simulink model "sampleModel20"  (R2021a)
settings: Solver=VariableStepAuto  StartTime=0.0  StopTime=10.0  RelTol=1e-3
undefined symbols (not defined in the file): DiscIntNeverNeededParam, magnitude, Newton, Raphson
libraries: simulink x274, pid_lib x17
(part 15 of 16)

== system sampleModel20/cfblk94/cfblk8/cfblk9/cfblk5 ==
  cfblk1 : Inport
  cfblk6 : Inport  Port=2
  cfblk7 : Inport  Port=3
  cfblk8 : Inport  Port=4
  cfblk9 : Inport  Port=5
  cfblk10 : Inport  Port=6
  cfblk3 : Assignment  DiagnosticForDimensions=Warning  IndexOptions=Index vector (dialog)  Indices=1  OutputSizes=1
  cfblk4 : Sin  TimeSource=Use external signal  SampleTime=0
  cfblk5 : Sum  Inputs=+-
  cfblk2 : Outport
  cfblk11 : Outport  Port=2
  wires:
  cfblk10/1 -> cfblk4/1
  cfblk1/1 -> cfblk2/1
  cfblk8/1 -> cfblk11/1
  cfblk9/1 -> cfblk5/1
  cfblk4/1 -> cfblk3/1
  cfblk7/1 -> cfblk3/2
  cfblk3/1 -> cfblk5/2

== system sampleModel20/cfblk94/cfblk9/cfblk6/cfblk10 ==
  cfblk1 : Inport
  cfblk3 : Inport  Port=2
  cfblk4 : Inport  Port=3
  cfblk5 : Inport  Port=4
  cfblk6 : Inport  Port=5
  cfblk7 : Inport  Port=6
  cfblk8 : Inport  Port=7
  cfblk9 : Inport  Port=8
  cfblk10 : Inport  Port=9
  cfblk11 : Inport  Port=10
  cfblk2 : Outport
  cfblk12 : Outport  Port=2
  cfblk13 : Outport  Port=3
  cfblk14 : Outport  Port=4
  wires:
  cfblk10/1 -> cfblk2/1
  cfblk6/1 -> cfblk12/1
  cfblk11/1 -> cfblk14/1
  cfblk7/1 -> cfblk13/1

== system sampleModel20/cfblk94/cfblk9/cfblk6/cfblk8 ==
  cfblk1 : Inport
  cfblk9 : Inport  Port=2
  cfblk10 : Inport  Port=3
  cfblk11 : Inport  Port=4
  cfblk12 : Inport  Port=5
  cfblk14 : Delay  SampleTime=1
  cfblk3 : Sqrt  Operator=rSqrt  AlgorithmType=Newton-Raphson  SaturateOnIntegerOverflow=on
  cfblk4 : Product
  cfblk5 : Sum  Inputs=+-
  cfblk6 : Math  SaturateOnIntegerOverflow=on
  cfblk7 : Abs
  cfblk8 : Sum  Inputs=+-
  cfblk2 : Outport
  cfblk13 : Outport  Port=2
  wires:
  cfblk8/1 -> cfblk7/1
  cfblk6/1 -> cfblk5/2
  cfblk5/1 -> cfblk4/1
  cfblk1/1 -> cfblk6/1
  cfblk12/1 -> cfblk3/1
  cfblk10/1 -> cfblk4/2
  cfblk3/1 -> cfblk8/1
  cfblk11/1 -> cfblk8/2
  cfblk7/1 -> cfblk13/1
  cfblk9/1 -> cfblk2/1
  cfblk4/1 -> cfblk14/1
  cfblk14/1 -> cfblk5/1

== system sampleModel20/cfblk94/cfblk9/cfblk6/cfblk9 ==
  cfblk1 : Inport
  cfblk7 : Inport  Port=2
  cfblk8 : Inport  Port=3
  cfblk9 : Inport  Port=4
  cfblk12 : Delay  SampleTime=1
  cfblk3 : Assignment  DiagnosticForDimensions=Warning  IndexOptions=Index vector (dialog)  Indices=1  OutputSizes=1
  cfblk4 : DotProduct  InputSameDT=on  OutDataTypeStr=Inherit: Inherit via internal rule
  cfblk5 : Sum  Inputs=|++
  cfblk6 : Math  Operator=log  SaturateOnIntegerOverflow=on
  cfblk2 : Outport
  cfblk10 : Outport  Port=2
  cfblk11 : Outport  Port=3
  wires:
  cfblk9/1 -> cfblk6/1
  cfblk8/1 -> cfblk11/1
  cfblk5/1 -> cfblk10/1, cfblk4/2, cfblk3/2
  cfblk1/1 -> cfblk5/2
  cfblk6/1 -> cfblk4/1
  cfblk7/1 -> cfblk3/1
  cfblk4/1 -> cfblk2/1
  cfblk3/1 -> cfblk12/1
  cfblk12/1 -> cfblk5/1

== system sampleModel20/cfblk95/cfblk10/cfblk7/cfblk7 ==
  cfblk1 : Inport
  cfblk7 : Inport  Port=2
  cfblk3 : Sum  Inputs=+
  cfblk4 : MinMax
  cfblk5 : Sqrt  SaturateOnIntegerOverflow=on
  cfblk6 : Bias  Bias=[-377808434.956185]
  cfblk8 : Delay  SampleTime=1
  cfblk2 : Outport
  wires:
  cfblk6/1 -> cfblk4/1
  cfblk3/1 -> cfblk5/1
  cfblk1/1 -> cfblk2/1
  cfblk5/1 -> cfblk6/1
  cfblk4/1 -> cfblk8/1
  cfblk8/1 -> cfblk3/1

== system sampleModel20/cfblk95/cfblk10/cfblk7/cfblk8 ==
  cfblk1 : Inport
  cfblk6 : Inport  Port=2
  cfblk7 : Inport  Port=3
  cfblk8 : Inport  Port=4
  cfblk9 : Inport  Port=5
  cfblk10 : Delay  SampleTime=1
  cfblk3 : Gain  Gain=[-39886875.988626]
  cfblk4 : ComplexToMagnitudeAngle
  cfblk5 : Reshape
  cfblk2 : Outport
  wires:
  cfblk3/1 -> cfblk4/1
  cfblk4/2 -> cfblk5/1
  cfblk7/1 -> cfblk2/1
  cfblk4/1 -> cfblk10/1
  cfblk10/1 -> cfblk3/1

== system sampleModel20/cfblk95/cfblk10/cfblk7/cfblk9 ==
  cfblk1 : Inport
  cfblk8 : Inport  Port=2
  cfblk9 : Inport  Port=3
  cfblk10 : Inport  Port=4
  cfblk11 : Inport  Port=5
  cfblk13 : Delay  SampleTime=1
  cfblk3 : Product
  cfblk4 : Sin  TimeSource=Use external signal  SampleTime=0
  cfblk5 : simulink/Math Operations/Slider Gain  gain=1  low=0  high=2
  cfblk6 : simulink/Math Operations/Slider Gain  gain=1  low=0  high=2
  cfblk7 : Product
  cfblk2 : Outport
  cfblk12 : Outport  Port=2
  wires:
  cfblk10/1 -> cfblk3/1
  cfblk8/1 -> cfblk7/1
  cfblk3/1 -> cfblk2/1
  cfblk1/1 -> cfblk5/1
  cfblk4/1 -> cfblk7/2
  cfblk7/1 -> cfblk6/1
  cfblk11/1 -> cfblk3/2
  cfblk5/1 -> cfblk12/1
  cfblk6/1 -> cfblk13/1
  cfblk13/1 -> cfblk4/1

== system sampleModel20/cfblk95/cfblk11/cfblk5/cfblk7 ==
  cfblk1 : Inport
  cfblk7 : Inport  Port=2
  cfblk8 : Inport  Port=3
  cfblk9 : Inport  Port=4
  cfblk3 : ComplexToRealImag
  cfblk4 : Squeeze
  cfblk5 : UnaryMinus
  cfblk6 : Squeeze
  cfblk2 : Outport
  wires:
  cfblk1/1 -> cfblk2/1
  cfblk9/1 -> cfblk5/1
  cfblk8/1 -> cfblk6/1
  cfblk6/1 -> cfblk4/1
  cfblk5/1 -> cfblk3/1

== system sampleModel20/cfblk95/cfblk11/cfblk5/cfblk8 ==
  cfblk1 : Inport
  cfblk9 : Inport  Port=2
  cfblk10 : Inport  Port=3
  cfblk11 : Inport  Port=4
  cfblk12 : Inport  Port=5
  cfblk13 : Inport  Port=6
  cfblk16 : Delay  SampleTime=1
  cfblk3 : Product  Inputs=*
  cfblk4 : Assignment  DiagnosticForDimensions=Warning  IndexOptions=Index vector (dialog)  Indices=1  OutputSizes=1
  cfblk5 : UnaryMinus
  cfblk6 : MinMax  Inputs=3
  cfblk7 : Sqrt  SaturateOnIntegerOverflow=on
  cfblk8 : ComplexToRealImag
  cfblk2 : Outport
  cfblk14 : Outport  Port=2
  cfblk15 : Outport  Port=3
  wires:
  cfblk7/1 -> cfblk15/1
  cfblk11/1 -> cfblk14/1
  cfblk6/1 -> cfblk5/1
  cfblk8/1 -> cfblk4/1
  cfblk10/1 -> cfblk7/1
  cfblk8/2 -> cfblk6/1
  cfblk13/1 -> cfblk3/1
  cfblk1/1 -> cfblk4/2
  cfblk9/1 -> cfblk2/1
  cfblk3/1 -> cfblk8/1
  cfblk12/1 -> cfblk6/3
  cfblk5/1 -> cfblk16/1
  cfblk16/1 -> cfblk6/2

== system sampleModel20/cfblk95/cfblk11/cfblk5/cfblk9 ==
  cfblk1 : Inport
  cfblk8 : Inport  Port=2
  cfblk9 : Inport  Port=3
  cfblk10 : Inport  Port=4
  cfblk11 : Inport  Port=5
  cfblk3 : Sqrt  SaturateOnIntegerOverflow=on
  cfblk4 : Gain  Gain=[617379721.728358]
  cfblk5 : Reshape
  cfblk6 : simulink/Math Operations/MinMax Running Resettable  Function=min  vinit=0.0
  cfblk7 : Bias  Bias=[626466756.933337]
  cfblk2 : Outport
  cfblk12 : Outport  Port=2
  wires:
  cfblk4/1 -> cfblk5/1
  cfblk6/1 -> cfblk7/1
  cfblk11/1 -> cfblk2/1
  cfblk8/1 -> cfblk4/1
  cfblk5/1 -> cfblk3/1
  cfblk3/1 -> cfblk12/1
  cfblk9/1 -> cfblk6/1
  cfblk1/1 -> cfblk6/2

== system sampleModel20/cfblk95/cfblk11/cfblk6/cfblk3 ==
  cfblk1 : Inport
  cfblk9 : Inport  Port=2
  cfblk11 : Delay  SampleTime=1
  cfblk3 : Rounding
  cfblk4 : ComplexToRealImag
  cfblk5 : DotProduct  InputSameDT=on  OutDataTypeStr=Inherit: Inherit via internal rule
  cfblk6 : MinMax  Inputs=2
  cfblk7 : Sqrt  Operator=rSqrt  AlgorithmType=Newton-Raphson  SaturateOnIntegerOverflow=on
  cfblk8 : DotProduct  InputSameDT=on  OutDataTypeStr=Inherit: Inherit via internal rule
  cfblk2 : Outport
  cfblk10 : Outport  Port=2
  wires:
  cfblk9/1 -> cfblk4/1
  cfblk4/1 -> cfblk8/1
  cfblk8/1 -> cfblk6/2, cfblk11/1
  cfblk6/1 -> cfblk10/1
  cfblk5/1 -> cfblk8/2
  cfblk1/1 -> cfblk7/1
  cfblk7/1 -> cfblk3/1
  cfblk4/2 -> cfblk6/1, cfblk2/1
  cfblk3/1 -> cfblk5/2
  cfblk11/1 -> cfblk5/1

== system sampleModel20/cfblk95/cfblk11/cfblk6/cfblk4 ==
  cfblk1 : Inport
  cfblk7 : Inport  Port=2
  cfblk8 : Inport  Port=3
  cfblk9 : Inport  Port=4
  cfblk10 : Inport  Port=5
  cfblk14 : Delay  SampleTime=1
  cfblk3 : Product  Inputs=**
  cfblk4 : Math  Operator=hypot  SaturateOnIntegerOverflow=on
  cfblk5 : Squeeze
  cfblk6 : Sum  Inputs=+-
  cfblk2 : Outport
  cfblk11 : Outport  Port=2
  cfblk12 : Outport  Port=3
  cfblk13 : Outport  Port=4
  wires:
  cfblk4/1 -> cfblk5/1
  cfblk6/1 -> cfblk12/1
  cfblk10/1 -> cfblk3/1, cfblk4/1
  cfblk5/1 -> cfblk13/1, cfblk14/1
  cfblk1/1 -> cfblk2/1
  cfblk8/1 -> cfblk11/1
  cfblk7/1 -> cfblk3/2
  cfblk9/1 -> cfblk6/1
  cfblk3/1 -> cfblk6/2
  cfblk14/1 -> cfblk4/2

== system sampleModel20/cfblk95/cfblk6/cfblk5/cfblk10 ==
  cfblk1 : Inport
  cfblk8 : Inport  Port=2
  cfblk9 : Inport  Port=3
  cfblk3 : Sum  Inputs=+
  cfblk4 : Sqrt  SaturateOnIntegerOverflow=on
  cfblk5 : Trigonometry
  cfblk6 : Product  Inputs=*
  cfblk7 : Constant  Value=[-128317265.699425]  SampleTime=1
  cfblk2 : Outport
  cfblk10 : Outport  Port=2
  cfblk11 : Outport  Port=3
  cfblk12 : Outport  Port=4
  cfblk13 : Outport  Port=5
  cfblk14 : Outport  Port=6
  wires:
  cfblk7/1 -> cfblk12/1
  cfblk1/1 -> cfblk10/1, cfblk11/1
  cfblk9/1 -> cfblk13/1
  cfblk8/1 -> cfblk4/1
  cfblk6/1 -> cfblk14/1
  cfblk4/1 -> cfblk3/1
  cfblk5/1 -> cfblk2/1, cfblk6/1
  cfblk3/1 -> cfblk5/1

== system sampleModel20/cfblk95/cfblk6/cfblk5/cfblk8 ==
  cfblk1 : Inport
  cfblk10 : Inport  Port=2
  cfblk11 : Inport  Port=3
  cfblk12 : Inport  Port=4
  cfblk13 : Inport  Port=5
  cfblk14 : Inport  Port=6
  cfblk15 : Inport  Port=7
  cfblk16 : Inport  Port=8
  cfblk3 : Math  Operator=conj  SaturateOnIntegerOverflow=on
  cfblk4 : Sin  TimeSource=Use external signal  SampleTime=0
  cfblk5 : simulink/Math Operations/Slider Gain  gain=1  low=0  high=2
  cfblk6 : ComplexToRealImag
  cfblk7 : Sum  Inputs=+-
  cfblk8 : Sqrt  SaturateOnIntegerOverflow=on
  cfblk9 : Squeeze
  cfblk2 : Outport
  cfblk17 : Outport  Port=2
  wires:
  cfblk1/1 -> cfblk3/1
  cfblk12/1 -> cfblk8/1
  cfblk16/1 -> cfblk4/1
  cfblk15/1 -> cfblk5/1
  cfblk4/1 -> cfblk9/1
  cfblk10/1 -> cfblk6/1
  cfblk11/1 -> cfblk2/1
  cfblk7/1 -> cfblk17/1
  cfblk9/1 -> cfblk7/1
  cfblk8/1 -> cfblk7/2

== system sampleModel20/cfblk95/cfblk6/cfblk5/cfblk9 ==
  cfblk1 : Inport
  cfblk10 : Inport  Port=2
  cfblk11 : Inport  Port=3
  cfblk12 : Inport  Port=4
  cfblk13 : Inport  Port=5
  cfblk14 : Inport  Port=6
  cfblk15 : Inport  Port=7
  cfblk3 : Reshape
  cfblk4 : simulink/Math Operations/Slider Gain  gain=1  low=0  high=2
  cfblk5 : Reshape
  cfblk6 : UnaryMinus
  cfblk7 : Sum  Inputs=|++
  cfblk8 : Abs
  cfblk9 : simulink/Math Operations/MinMax Running Resettable  Function=min  vinit=0.0
  cfblk2 : Outport
  cfblk16 : Outport  Port=2
  cfblk17 : Outport  Port=3
  wires:
  cfblk11/1 -> cfblk9/1
  cfblk8/1 -> cfblk6/1
  cfblk3/1 -> cfblk8/1
  cfblk4/1 -> cfblk5/1
  cfblk7/1 -> cfblk4/1
  cfblk1/1 -> cfblk7/1
  cfblk15/1 -> cfblk9/2
  cfblk10/1 -> cfblk17/1
  cfblk14/1 -> cfblk7/2
  cfblk13/1 -> cfblk16/1
  cfblk6/1 -> cfblk2/1
  cfblk9/1 -> cfblk3/1

== system sampleModel20/cfblk95/cfblk6/cfblk6/cfblk10 ==
  cfblk1 : Inport
  cfblk6 : Inport  Port=2
  cfblk7 : Inport  Port=3
  cfblk8 : Inport  Port=4
  cfblk9 : Inport  Port=5
  cfblk10 : Inport  Port=6
  cfblk3 : DiscreteFir  SampleTime=1
  cfblk4 : UnaryMinus
  cfblk5 : Sum  Inputs=|++
  cfblk2 : Outport
  cfblk11 : Outport  Port=2
  wires:
  cfblk7/1 -> cfblk5/1
  cfblk9/1 -> cfblk2/1
  cfblk3/1 -> cfblk4/1
  cfblk6/1 -> cfblk5/2
  cfblk1/1 -> cfblk3/1
  cfblk5/1 -> cfblk11/1

== system sampleModel20/cfblk95/cfblk6/cfblk6/cfblk8 ==
  cfblk1 : Inport
  cfblk7 : Inport  Port=2
  cfblk8 : Inport  Port=3
  cfblk9 : Inport  Port=4
  cfblk10 : Delay  SampleTime=1
  cfblk3 : DiscreteTransferFcn  SampleTime=1
  cfblk4 : Sum  Inputs=+-
  cfblk5 : Gain  Gain=[-981035037.304290]
  cfblk6 : Product  Inputs=**
  cfblk2 : Outport
  wires:
  cfblk9/1 -> cfblk2/1
  cfblk6/1 -> cfblk5/1
  cfblk8/1 -> cfblk4/1
  cfblk3/1 -> cfblk6/1
  cfblk7/1 -> cfblk6/2
  cfblk1/1 -> cfblk4/2
  cfblk5/1 -> cfblk10/1
  cfblk10/1 -> cfblk3/1

== system sampleModel20/cfblk95/cfblk6/cfblk6/cfblk9 ==
  cfblk1 : Inport
  cfblk9 : Inport  Port=2
  cfblk10 : Inport  Port=3
  cfblk11 : Inport  Port=4
  cfblk12 : Inport  Port=5
  cfblk3 : Gain  Gain=[466248434.807061]
  cfblk4 : Trigonometry
  cfblk5 : Signum
  cfblk6 : Rounding
  cfblk7 : Squeeze
  cfblk8 : Sum  Inputs=+
  cfblk2 : Outport
  cfblk13 : Outport  Port=2
  wires:
  cfblk4/1 -> cfblk2/1
  cfblk9/1 -> cfblk6/1
  cfblk6/1 -> cfblk3/1
  cfblk10/1 -> cfblk4/1
  cfblk3/1 -> cfblk5/1
  cfblk1/1 -> cfblk7/1
  cfblk11/1 -> cfblk8/1
  cfblk12/1 -> cfblk13/1

== system sampleModel20/cfblk95/cfblk6/cfblk7/cfblk10 ==
  cfblk1 : Inport
  cfblk10 : Inport  Port=2
  cfblk11 : Inport  Port=3
  cfblk12 : Inport  Port=4
  cfblk13 : Inport  Port=5
  cfblk14 : Inport  Port=6
  cfblk15 : Inport  Port=7
  cfblk3 : Sqrt  Operator=rSqrt  AlgorithmType=Newton-Raphson  SaturateOnIntegerOverflow=on
  cfblk4 : Sum  Inputs=|++
  cfblk5 : Sum  Inputs=+
  cfblk6 : Signum
  cfblk7 : Gain  Gain=[306381383.293129]
  cfblk8 : Gain  Gain=[360787221.537150]
  cfblk9 : Polyval  Coefs=[ +2.081618890e-019, -1.441693666e-014, +4.719686976e-010, -8.536869453e-006, +1.621573104e-001, -8.087801117e+001 ]
  cfblk2 : Outport
  cfblk16 : Outport  Port=2
  wires:
  cfblk11/1 -> cfblk7/1
  cfblk15/1 -> cfblk3/1
  cfblk7/1 -> cfblk5/1
  cfblk14/1 -> cfblk8/1
  cfblk9/1 -> cfblk4/1
  cfblk1/1 -> cfblk9/1
  cfblk3/1 -> cfblk16/1
  cfblk13/1 -> cfblk6/1
  cfblk6/1 -> cfblk4/2
  cfblk4/1 -> cfblk2/1

== system sampleModel20/cfblk95/cfblk6/cfblk7/cfblk11 ==
  cfblk1 : Inport
  cfblk5 : Inport  Port=2
  cfblk6 : Inport  Port=3
  cfblk7 : Inport  Port=4
  cfblk8 : Inport  Port=5
  cfblk9 : Inport  Port=6
  cfblk3 : DiscreteFir  SampleTime=1
  cfblk4 : Sum  Inputs=-+
  cfblk2 : Outport
  cfblk10 : Outport  Port=2
  wires:
  cfblk8/1 -> cfblk10/1
  cfblk6/1 -> cfblk2/1
  cfblk5/1 -> cfblk3/1
  cfblk1/1 -> cfblk4/1
  cfblk7/1 -> cfblk4/2

== system sampleModel20/cfblk95/cfblk6/cfblk7/cfblk9 ==
  cfblk1 : Inport
  cfblk5 : Inport  Port=2
  cfblk6 : Inport  Port=3
  cfblk7 : Inport  Port=4
  cfblk3 : Sqrt  Operator=rSqrt  AlgorithmType=Newton-Raphson  SaturateOnIntegerOverflow=on
  cfblk4 : Squeeze
  cfblk2 : Outport
  wires:
  cfblk3/1 -> cfblk4/1
  cfblk1/1 -> cfblk3/1
  cfblk6/1 -> cfblk2/1

== system sampleModel20/cfblk95/cfblk7/cfblk4/cfblk10 ==
  cfblk1 : Inport
  cfblk8 : Inport  Port=2
  cfblk9 : Inport  Port=3
  cfblk10 : Inport  Port=4
  cfblk11 : Inport  Port=5
  cfblk12 : Inport  Port=6
  cfblk13 : Inport  Port=7
  cfblk3 : DiscreteZeroPole  Poles=[0 0.5]  Gain=1
  cfblk4 : Signum
  cfblk5 : Signum
  cfblk6 : simulink/Math Operations/Slider Gain  gain=1  low=0  high=2
  cfblk7 : Assignment  DiagnosticForDimensions=Warning  IndexOptions=Index vector (dialog)  Indices=1  OutputSizes=1
  cfblk2 : Outport
  cfblk14 : Outport  Port=2
  cfblk15 : Outport  Port=3
  cfblk16 : Outport  Port=4
  cfblk17 : Outport  Port=5
  wires:
  cfblk1/1 -> cfblk3/1
  cfblk7/1 -> cfblk16/1
  cfblk12/1 -> cfblk4/1
  cfblk3/1 -> cfblk5/1
  cfblk6/1 -> cfblk14/1
  cfblk11/1 -> cfblk15/1
  cfblk13/1 -> cfblk6/1
  cfblk8/1 -> cfblk2/1
  cfblk10/1 -> cfblk7/1
  cfblk5/1 -> cfblk17/1
  cfblk9/1 -> cfblk7/2

== system sampleModel20/cfblk95/cfblk7/cfblk4/cfblk7 ==
  cfblk1 : Inport
  cfblk7 : Inport  Port=2
  cfblk8 : Inport  Port=3
  cfblk9 : Inport  Port=4
  cfblk10 : Inport  Port=5
  cfblk11 : Inport  Port=6
  cfblk3 : DotProduct  InputSameDT=on  OutDataTypeStr=Inherit: Inherit via internal rule
  cfblk4 : ComplexToMagnitudeAngle
  cfblk5 : Sqrt  SaturateOnIntegerOverflow=on
  cfblk6 : Bias  Bias=[-832558987.435364]
  cfblk2 : Outport
  wires:
  cfblk11/1 -> cfblk6/1
  cfblk9/1 -> cfblk5/1
  cfblk5/1 -> cfblk3/1
  cfblk6/1 -> cfblk4/1
  cfblk7/1 -> cfblk2/1
  cfblk1/1 -> cfblk3/2

== system sampleModel20/cfblk95/cfblk7/cfblk4/cfblk8 ==
  cfblk1 : Inport
  cfblk8 : Inport  Port=2
  cfblk9 : Inport  Port=3
  cfblk10 : Inport  Port=4
  cfblk12 : Delay  SampleTime=1
  cfblk3 : Product  Inputs=**
  cfblk4 : Product  Inputs=*
  cfblk5 : Assignment  DiagnosticForDimensions=Warning  IndexOptions=Index vector (dialog)  Indices=1  OutputSizes=1
  cfblk6 : Signum
  cfblk7 : ComplexToRealImag
  cfblk2 : Outport
  cfblk11 : Outport  Port=2
  wires:
  cfblk3/1 -> cfblk5/1
  cfblk7/1 -> cfblk2/1
  cfblk8/1 -> cfblk7/1
  cfblk4/1 -> cfblk6/1
  cfblk10/1 -> cfblk5/2
  cfblk6/1 -> cfblk3/1
  cfblk7/2 -> cfblk11/1
  cfblk9/1 -> cfblk4/1
  cfblk5/1 -> cfblk12/1
  cfblk12/1 -> cfblk3/2

== system sampleModel20/cfblk95/cfblk7/cfblk4/cfblk9 ==
  cfblk1 : Inport
  cfblk8 : Inport  Port=2
  cfblk9 : Inport  Port=3
  cfblk10 : Inport  Port=4
  cfblk11 : Inport  Port=5
  cfblk12 : Inport  Port=6
  cfblk13 : Inport  Port=7
  cfblk14 : Inport  Port=8
  cfblk15 : Inport  Port=9
  cfblk3 : Product
  cfblk4 : Squeeze
  cfblk5 : Gain  Gain=[-607601415.190912]
  cfblk6 : Sqrt  Operator=rSqrt  AlgorithmType=Newton-Raphson  SaturateOnIntegerOverflow=on
  cfblk7 : Sum  Inputs=|++
  cfblk2 : Outport
  cfblk16 : Outport  Port=2
  cfblk17 : Outport  Port=3
  wires:
  cfblk13/1 -> cfblk3/1
  cfblk1/1 -> cfblk2/1
  cfblk5/1 -> cfblk4/1
  cfblk8/1 -> cfblk3/2
  cfblk3/1 -> cfblk16/1
  cfblk12/1 -> cfblk7/1
  cfblk11/1 -> cfblk6/1
  cfblk10/1 -> cfblk5/1
  cfblk15/1 -> cfblk7/2
  cfblk6/1 -> cfblk17/1

== system sampleModel20/cfblk95/cfblk7/cfblk5/cfblk5 ==
  cfblk1 : Inport
  cfblk8 : Inport  Port=2
  cfblk9 : Inport  Port=3
  cfblk10 : Inport  Port=4
  cfblk11 : Inport  Port=5
  cfblk12 : Inport  Port=6
  cfblk13 : Inport  Port=7
  cfblk3 : Trigonometry
  cfblk4 : Rounding
  cfblk5 : Product  Inputs=*
  cfblk6 : Sum  Inputs=+
  cfblk7 : Bias  Bias=[7544371.350967]
  cfblk2 : Outport
  cfblk14 : Outport  Port=2
  cfblk15 : Outport  Port=3
  wires:
  cfblk1/1 -> cfblk5/1
  cfblk10/1 -> cfblk2/1
  cfblk3/1 -> cfblk7/1
  cfblk9/1 -> cfblk6/1
  cfblk8/1 -> cfblk14/1
  cfblk11/1 -> cfblk3/1
  cfblk13/1 -> cfblk4/1
  cfblk4/1 -> cfblk15/1

== system sampleModel20/cfblk95/cfblk7/cfblk5/cfblk6 ==
  cfblk1 : Inport
  cfblk5 : Inport  Port=2
  cfblk6 : Inport  Port=3
  cfblk7 : Inport  Port=4
  cfblk3 : Product  Inputs=**
  cfblk4 : UnaryMinus
  cfblk2 : Outport
  cfblk8 : Outport  Port=2
  wires:
  cfblk5/1 -> cfblk4/1
  cfblk3/1 -> cfblk8/1
  cfblk1/1 -> cfblk2/1
  cfblk7/1 -> cfblk3/1
  cfblk6/1 -> cfblk3/2

== system sampleModel20/cfblk95/cfblk8/cfblk5/cfblk6 ==
  cfblk1 : Inport
  cfblk6 : Inport  Port=2
  cfblk7 : Inport  Port=3
  cfblk8 : Inport  Port=4
  cfblk3 : Sum  Inputs=|++
  cfblk4 : Gain  Gain=[-834854673.275591]
  cfblk5 : Sum  Inputs=+-
  cfblk2 : Outport
  cfblk9 : Outport  Port=2
  cfblk10 : Outport  Port=3
  wires:
  cfblk7/1 -> cfblk3/1
  cfblk3/1 -> cfblk10/1
  cfblk5/1 -> cfblk3/2
  cfblk8/1 -> cfblk9/1
  cfblk1/1 -> cfblk2/1
  cfblk6/1 -> cfblk4/1, cfblk5/2
  cfblk4/1 -> cfblk5/1

== system sampleModel20/cfblk95/cfblk8/cfblk6/cfblk10 ==
  cfblk1 : Inport
  cfblk5 : Inport  Port=2
  cfblk6 : Inport  Port=3
  cfblk7 : Inport  Port=4
  cfblk8 : Inport  Port=5
  cfblk3 : Sqrt  Operator=rSqrt  AlgorithmType=Newton-Raphson  SaturateOnIntegerOverflow=on
  cfblk4 : Sum  Inputs=+-
  cfblk2 : Outport
  wires:
  cfblk6/1 -> cfblk3/1
  cfblk7/1 -> cfblk2/1
  cfblk1/1 -> cfblk4/1
  cfblk8/1 -> cfblk4/2

== system sampleModel20/cfblk95/cfblk8/cfblk6/cfblk11 ==
  cfblk1 : Inport
  cfblk4 : Inport  Port=2
  cfblk5 : Inport  Port=3
  cfblk6 : Inport  Port=4
  cfblk3 : Sqrt  SaturateOnIntegerOverflow=on
  cfblk2 : Outport
  cfblk7 : Outport  Port=2
  wires:
  cfblk1/1 -> cfblk3/1
  cfblk4/1 -> cfblk7/1
  cfblk5/1 -> cfblk2/1

== system sampleModel20/cfblk95/cfblk8/cfblk6/cfblk12 ==
  cfblk1 : Inport
  cfblk9 : Inport  Port=2
  cfblk10 : Inport  Port=3
  cfblk11 : Inport  Port=4
  cfblk12 : Inport  Port=5
  cfblk13 : Inport  Port=6
  cfblk14 : Delay  SampleTime=1
  cfblk3 : MinMax  Function=max
  cfblk4 : PermuteDimensions
  cfblk5 : Sin  TimeSource=Use external signal  SampleTime=0
  cfblk6 : PermuteDimensions
  cfblk7 : Product
  cfblk8 : DotProduct  InputSameDT=on  OutDataTypeStr=Inherit: Inherit via internal rule
  cfblk2 : Outport
  wires:
  cfblk8/1 -> cfblk4/1
  cfblk11/1 -> cfblk2/1
  cfblk13/1 -> cfblk7/1
  cfblk5/1 -> cfblk6/1
  cfblk1/1 -> cfblk8/1
  cfblk12/1 -> cfblk7/2
  cfblk10/1 -> cfblk8/2
  cfblk7/1 -> cfblk3/1
  cfblk6/1 -> cfblk14/1
  cfblk14/1 -> cfblk5/1

== system sampleModel20/cfblk95/cfblk8/cfblk6/cfblk7 ==
  cfblk1 : Inport
  cfblk5 : Inport  Port=2
  cfblk6 : Inport  Port=3
  cfblk7 : Inport  Port=4
  cfblk3 : pid_lib/PID Controller (2DOF)  Controller=PID  Form=Parallel  TimeDomain=Discrete-time  UseExternalTs=off  SampleTime=1  IntegratorMethod=Forward Euler  FilterMethod=Forward Euler  ControllerParametersSource=internal  P=1  I=1  D=0  UseFilter=on  N=100  b=1  c=1  TunerSelectOption=Transfer Function Based (PID Tuner App)  InitialConditionSource=internal  InitialConditionForIntegrator=0  InitialConditionForFilter=0  DifferentiatorICPrevScaledInput=0  ExternalReset=none  TrackingMode=off  Kt=1  LimitOutput=off  SatLimitsSource=internal  UpperSaturationLimit=inf  LowerSaturationLimit=-inf  LinearizeAsGain=off  AntiWindupMode=none  Kb=1  POutMin=[]  POutMax=[]  IOutMin=[]  IOutMax=[]  DOutMin=[]  DOutMax=[]  NOutMin=[]  NOutMax=[]  bOutMin=[]  bOutMax=[]  cOutMin=[]  cOutMax=[]  SumOutMin=[]  SumOutMax=[]  SaturationOutMin=[]  SaturationOutMax=[]  PParamMin=[]  PParamMax=[]  IParamMin=[]  IParamMax=[]  DParamMin=[]  DParamMax=[]  NParamMin=[]  NParamMax=[]  bParamMin=[]  bParamMax=[]  cParamMin=[]  cParamMax=[]  KbParamMin=[]  KbParamMax=[]  KtParamMin=[]  KtParamMax=[]  KbOutMin=[]  KbOutMax=[]  KtOutMin=[]  KtOutMax=[]  IntegratorOutMin=[]  IntegratorOutMax=[]  FilterOutMin=[]  FilterOutMax=[]  SumI1OutMin=[]  SumI1OutMax=[]  SumI2OutMin=[]  SumI2OutMax=[]  SumI3OutMin=[]  SumI3OutMax=[]  SumI4OutMin=[]  SumI4OutMax=[]  SumDOutMin=[]  SumDOutMax=[]  Sum1OutMin=[]  Sum1OutMax=[]  Sum2OutMin=[]  Sum2OutMax=[]  Sum3OutMin=[]  Sum3OutMax=[]  DifferentiatorOutMin=[]  DifferentiatorOutMax=[]  FilterDiffOutCoefMin=[]  FilterDiffOutCoefMax=[]  ReciprocalOutMin=[]  ReciprocalOutMax=[]  SumDenOutMin=[]  SumDenOutMax=[]  SumNumOutMin=[]  SumNumOutMax=[]  DivideOutMin=[]  DivideOutMax=[]  UdiffTsProdOutMin=[]  UdiffTsProdOutMax=[]  NTsProdOutMin=[]  NTsProdOutMax=[]  UintegralTsProdOutMin=[]  UintegralTsProdOutMax=[]  UngainTsProdOutMin=[]  UngainTsProdOutMax=[]  IntegratorContinuousStateAttributes=''  IntegratorStateMustResolveToSignalObject=off  IntegratorRTWStateStorageClass=Auto  FilterContinuousStateAttributes=''  FilterStateMustResolveToSignalObject=off  FilterRTWStateStorageClass=Auto  ParallelPVariant=InternalParameters  IdealPVariant=Disabled  IVariant=InternalParameters  DVariant=InternalParameters  bVariant=InternalParameters  cVariant=InternalParameters  IntegratorVariant=Discrete  SatVariant=Disabled  AWVariant=Passthrough  PCopyVariant=Disabled  TRVariant=Disabled  FdbkBlocksVariant=Forward  IdealPFdbkVariant=Disabled  SatFdbkVariant=Disabled  DerivativeFilterVariant=ForwardEulerFilter  NVariant=InternalParameters  NCopyVariant=Disabled  FilterICVariant=InternalICsFilter  IntegratorICVariant=InternalICs  ExternalResetVariant=Disabled  TRSumVariant=Passthrough  SumFdbkVariant=Disabled  SumVariant=Sum_PID  TsampFilterVariant=InternalTs  TsampNgainVariant=Passthrough  TsampIntegralVariant=Passthrough  ExternalSaturationOutDataTypeStr=Inherit: Same as second input
      settings: SourceProductBaseCode=SL
  cfblk4 : Sqrt  Operator=rSqrt  AlgorithmType=Newton-Raphson  SaturateOnIntegerOverflow=on
  cfblk2 : Outport
  cfblk8 : Outport  Port=2
  cfblk9 : Outport  Port=3
  wires:
  cfblk6/1 -> cfblk4/1
  cfblk7/1 -> cfblk9/1
  cfblk4/1 -> cfblk2/1
  cfblk1/1 -> cfblk3/1
  cfblk3/1 -> cfblk8/1
  cfblk5/1 -> cfblk3/2

== system sampleModel20/cfblk95/cfblk8/cfblk6/cfblk8 ==
  cfblk1 : Inport
  cfblk10 : Inport  Port=2
  cfblk11 : Inport  Port=3
  cfblk12 : Inport  Port=4
  cfblk13 : Inport  Port=5
  cfblk14 : Inport  Port=6
  cfblk15 : Inport  Port=7
  cfblk3 : simulink/Discrete/Difference  ICPrevInput=0.0  OutMin=[]  OutMax=[]  OutDataTypeStr=Inherit: Inherit via back propagation  OutDataType=fixdt(1, 16)  OutScaling=2^-10  DoSatur=off
  cfblk4 : DotProduct  InputSameDT=on  OutDataTypeStr=Inherit: Inherit via internal rule
  cfblk5 : Reshape
  cfblk6 : simulink/Math Operations/Slider Gain  gain=1  low=0  high=2
  cfblk7 : Sin  TimeSource=Use external signal  SampleTime=0
  cfblk8 : UnaryMinus
  cfblk9 : Abs
  cfblk2 : Outport
  wires:
  cfblk3/1 -> cfblk6/1
  cfblk13/1 -> cfblk2/1
  cfblk7/1 -> cfblk9/1
  cfblk1/1 -> cfblk5/1
  cfblk9/1 -> cfblk8/1
  cfblk6/1 -> cfblk7/1
  cfblk11/1 -> cfblk3/1
  cfblk14/1 -> cfblk4/1
  cfblk15/1 -> cfblk4/2

== system sampleModel20/cfblk95/cfblk8/cfblk6/cfblk9 ==
  cfblk1 : Inport
  cfblk8 : Inport  Port=2
  cfblk9 : Inport  Port=3
  cfblk12 : Delay  SampleTime=1
  cfblk13 : Delay  SampleTime=1
  cfblk3 : DiscreteStateSpace
  cfblk4 : simulink/Math Operations/MinMax Running Resettable  Function=min  vinit=0.0
  cfblk5 : Product  Inputs=**
  cfblk6 : Gain  Gain=[-761792145.113436]
  cfblk7 : Sum  Inputs=+
  cfblk2 : Outport
  cfblk10 : Outport  Port=2
  cfblk11 : Outport  Port=3
  wires:
  cfblk4/1 -> cfblk10/1, cfblk5/2
  cfblk5/1 -> cfblk6/1, cfblk13/1
  cfblk8/1 -> cfblk11/1
  cfblk9/1 -> cfblk3/1
  cfblk6/1 -> cfblk7/1
  cfblk3/1 -> cfblk2/1
  cfblk1/1 -> cfblk4/1
  cfblk7/1 -> cfblk12/1
  cfblk12/1 -> cfblk5/1
  cfblk13/1 -> cfblk4/2

== system sampleModel20/cfblk95/cfblk8/cfblk7/cfblk5 ==
  cfblk1 : Inport
  cfblk6 : Inport  Port=2
  cfblk7 : Inport  Port=3
  cfblk8 : Inport  Port=4
  cfblk9 : Inport  Port=5
  cfblk10 : Inport  Port=6
  cfblk3 : Sum  Inputs=+-
  cfblk4 : Sum  Inputs=|++
  cfblk5 : Product
  cfblk2 : Outport
  wires:
  cfblk10/1 -> cfblk4/1
  cfblk9/1 -> cfblk3/1
  cfblk5/1 -> cfblk2/1
  cfblk1/1 -> cfblk3/2
  cfblk8/1 -> cfblk5/1
  cfblk3/1 -> cfblk4/2
  cfblk6/1 -> cfblk5/2

== system sampleModel20/cfblk95/cfblk8/cfblk7/cfblk6 ==
  cfblk1 : Inport
  cfblk12 : Inport  Port=2
  cfblk13 : Inport  Port=3
  cfblk14 : Inport  Port=4
  cfblk10 : Product  Inputs=*
  cfblk11 : Sin  TimeSource=Use external signal  SampleTime=0
  cfblk17 : Delay  SampleTime=1
  cfblk3 : Signum
  cfblk4 : Sum  Inputs=|++
  cfblk5 : Sum  Inputs=+
  cfblk6 : Sqrt  SaturateOnIntegerOverflow=on
  cfblk7 : Abs
  cfblk8 : Math  Operator=mod  SaturateOnIntegerOverflow=on
  cfblk9 : Trigonometry
  cfblk2 : Outport
  cfblk15 : Outport  Port=2
  cfblk16 : Outport  Port=3
  wires:
  cfblk10/1 -> cfblk8/1, cfblk2/1
  cfblk1/1 -> cfblk6/1
  cfblk8/1 -> cfblk4/1
  cfblk9/1 -> cfblk4/2
  cfblk14/1 -> cfblk10/1
  cfblk13/1 -> cfblk16/1
  cfblk12/1 -> cfblk3/1
  cfblk4/1 -> cfblk15/1
  cfblk7/1 -> cfblk9/1
  cfblk6/1 -> cfblk8/2
  cfblk5/1 -> cfblk11/1
  cfblk3/1 -> cfblk7/1
  cfblk11/1 -> cfblk17/1
  cfblk17/1 -> cfblk5/1

== system sampleModel20/cfblk95/cfblk8/cfblk7/cfblk7 ==
  cfblk1 : Inport
  cfblk9 : Inport  Port=2
  cfblk10 : Inport  Port=3
  cfblk11 : Inport  Port=4
  cfblk12 : Inport  Port=5
  cfblk13 : Inport  Port=6
  cfblk17 : Delay  SampleTime=1
  cfblk3 : pid_lib/PID Controller (2DOF)  Controller=PID  Form=Parallel  TimeDomain=Discrete-time  UseExternalTs=off  SampleTime=1  IntegratorMethod=Forward Euler  FilterMethod=Forward Euler  ControllerParametersSource=internal  P=1  I=1  D=0  UseFilter=on  N=100  b=1  c=1  TunerSelectOption=Transfer Function Based (PID Tuner App)  InitialConditionSource=internal  InitialConditionForIntegrator=0  InitialConditionForFilter=0  DifferentiatorICPrevScaledInput=0  ExternalReset=none  TrackingMode=off  Kt=1  LimitOutput=off  SatLimitsSource=internal  UpperSaturationLimit=inf  LowerSaturationLimit=-inf  LinearizeAsGain=off  AntiWindupMode=none  Kb=1  POutMin=[]  POutMax=[]  IOutMin=[]  IOutMax=[]  DOutMin=[]  DOutMax=[]  NOutMin=[]  NOutMax=[]  bOutMin=[]  bOutMax=[]  cOutMin=[]  cOutMax=[]  SumOutMin=[]  SumOutMax=[]  SaturationOutMin=[]  SaturationOutMax=[]  PParamMin=[]  PParamMax=[]  IParamMin=[]  IParamMax=[]  DParamMin=[]  DParamMax=[]  NParamMin=[]  NParamMax=[]  bParamMin=[]  bParamMax=[]  cParamMin=[]  cParamMax=[]  KbParamMin=[]  KbParamMax=[]  KtParamMin=[]  KtParamMax=[]  KbOutMin=[]  KbOutMax=[]  KtOutMin=[]  KtOutMax=[]  IntegratorOutMin=[]  IntegratorOutMax=[]  FilterOutMin=[]  FilterOutMax=[]  SumI1OutMin=[]  SumI1OutMax=[]  SumI2OutMin=[]  SumI2OutMax=[]  SumI3OutMin=[]  SumI3OutMax=[]  SumI4OutMin=[]  SumI4OutMax=[]  SumDOutMin=[]  SumDOutMax=[]  Sum1OutMin=[]  Sum1OutMax=[]  Sum2OutMin=[]  Sum2OutMax=[]  Sum3OutMin=[]  Sum3OutMax=[]  DifferentiatorOutMin=[]  DifferentiatorOutMax=[]  FilterDiffOutCoefMin=[]  FilterDiffOutCoefMax=[]  ReciprocalOutMin=[]  ReciprocalOutMax=[]  SumDenOutMin=[]  SumDenOutMax=[]  SumNumOutMin=[]  SumNumOutMax=[]  DivideOutMin=[]  DivideOutMax=[]  UdiffTsProdOutMin=[]  UdiffTsProdOutMax=[]  NTsProdOutMin=[]  NTsProdOutMax=[]  UintegralTsProdOutMin=[]  UintegralTsProdOutMax=[]  UngainTsProdOutMin=[]  UngainTsProdOutMax=[]  IntegratorContinuousStateAttributes=''  IntegratorStateMustResolveToSignalObject=off  IntegratorRTWStateStorageClass=Auto  FilterContinuousStateAttributes=''  FilterStateMustResolveToSignalObject=off  FilterRTWStateStorageClass=Auto  ParallelPVariant=InternalParameters  IdealPVariant=Disabled  IVariant=InternalParameters  DVariant=InternalParameters  bVariant=InternalParameters  cVariant=InternalParameters  IntegratorVariant=Discrete  SatVariant=Disabled  AWVariant=Passthrough  PCopyVariant=Disabled  TRVariant=Disabled  FdbkBlocksVariant=Forward  IdealPFdbkVariant=Disabled  SatFdbkVariant=Disabled  DerivativeFilterVariant=ForwardEulerFilter  NVariant=InternalParameters  NCopyVariant=Disabled  FilterICVariant=InternalICsFilter  IntegratorICVariant=InternalICs  ExternalResetVariant=Disabled  TRSumVariant=Passthrough  SumFdbkVariant=Disabled  SumVariant=Sum_PID  TsampFilterVariant=InternalTs  TsampNgainVariant=Passthrough  TsampIntegralVariant=Passthrough  ExternalSaturationOutDataTypeStr=Inherit: Same as second input
      settings: SourceProductBaseCode=SL
  cfblk4 : PermuteDimensions
  cfblk5 : Sum
  cfblk6 : Sum  Inputs=+
  cfblk7 : Squeeze
  cfblk8 : Bias  Bias=[-624899519.034354]
  cfblk2 : Outport
  cfblk14 : Outport  Port=2
  cfblk15 : Outport  Port=3
  cfblk16 : Outport  Port=4
  wires:
  cfblk8/1 -> cfblk14/1
  cfblk1/1 -> cfblk2/1
  cfblk5/1 -> cfblk6/1
  cfblk10/1 -> cfblk4/1
  cfblk12/1 -> cfblk3/1
  cfblk4/1 -> cfblk3/2
  cfblk9/1 -> cfblk16/1
  cfblk6/1 -> cfblk7/1
  cfblk13/1 -> cfblk15/1
  cfblk11/1 -> cfblk5/2
  cfblk3/1 -> cfblk8/1
  cfblk7/1 -> cfblk17/1
  cfblk17/1 -> cfblk5/1

== system sampleModel20/cfblk95/cfblk9/cfblk7/cfblk6 ==
  cfblk1 : Inport
  cfblk5 : Inport  Port=2
  cfblk6 : Inport  Port=3
  cfblk7 : Inport  Port=4
  cfblk8 : Inport  Port=5
  cfblk9 : Inport  Port=6
  cfblk10 : Inport  Port=7
  cfblk11 : Inport  Port=8
  cfblk12 : Inport  Port=9
  cfblk13 : Inport  Port=10
  cfblk14 : Inport  Port=11
  cfblk3 : Sqrt  Operator=rSqrt  AlgorithmType=Newton-Raphson  SaturateOnIntegerOverflow=on
  cfblk4 : ComplexToRealImag
  cfblk2 : Outport
  wires:
  cfblk9/1 -> cfblk2/1
  cfblk10/1 -> cfblk3/1
  cfblk11/1 -> cfblk4/1

== system sampleModel20/cfblk95/cfblk9/cfblk7/cfblk7 ==
  cfblk1 : Inport
  cfblk6 : Inport  Port=2
  cfblk7 : Inport  Port=3
  cfblk8 : Inport  Port=4
  cfblk3 : Signum
  cfblk4 : Sum  Inputs=+
  cfblk5 : MinMax  Function=max
  cfblk2 : Outport
  wires:
  cfblk5/1 -> cfblk2/1
  cfblk7/1 -> cfblk3/1
  cfblk8/1 -> cfblk4/1
  cfblk4/1 -> cfblk5/1

== system sampleModel20/cfblk95/cfblk9/cfblk8/cfblk7 ==
  cfblk1 : Inport
  cfblk7 : Inport  Port=2
  cfblk8 : Inport  Port=3
  cfblk9 : Inport  Port=4
  cfblk10 : Inport  Port=5
  cfblk3 : Sum  Inputs=|++
  cfblk4 : Product  Inputs=**
  cfblk5 : Product  Inputs=**
  cfblk6 : Rounding
  cfblk2 : Outport
  cfblk11 : Outport  Port=2
  cfblk12 : Outport  Port=3
  cfblk13 : Outport  Port=4
  wires:
  cfblk4/1 -> cfblk12/1
  cfblk8/1 -> cfblk5/1
  cfblk9/1 -> cfblk11/1
  cfblk7/1 -> cfblk2/1, cfblk3/2
  cfblk10/1 -> cfblk5/2
  cfblk6/1 -> cfblk4/1
  cfblk5/1 -> cfblk3/1, cfblk4/2
  cfblk3/1 -> cfblk6/1
  cfblk1/1 -> cfblk13/1

== system sampleModel20/cfblk96/cfblk5/cfblk4/cfblk10 ==
  cfblk1 : Inport
  cfblk8 : Inport  Port=2
  cfblk9 : Inport  Port=3
  cfblk10 : Inport  Port=4
  cfblk11 : Inport  Port=5
  cfblk3 : DotProduct  InputSameDT=on  OutDataTypeStr=Inherit: Inherit via internal rule
  cfblk4 : Product
  cfblk5 : Sin  TimeSource=Use external signal  SampleTime=0
  cfblk6 : ComplexToRealImag
  cfblk7 : Sum  Inputs=+-
  cfblk2 : Outport
  cfblk12 : Outport  Port=2
  cfblk13 : Outport  Port=3
  cfblk14 : Outport  Port=4
  cfblk15 : Outport  Port=5
  cfblk16 : Outport  Port=6
  wires:
  cfblk3/1 -> cfblk5/1
  cfblk9/1 -> cfblk6/1
  cfblk11/1 -> cfblk16/1
  cfblk1/1 -> cfblk15/1, cfblk12/1
  cfblk4/1 -> cfblk3/1
  cfblk6/1 -> cfblk3/2
  cfblk6/2 -> cfblk14/1
  cfblk7/1 -> cfblk2/1
  cfblk10/1 -> cfblk4/1, cfblk13/1, cfblk7/2
  cfblk8/1 -> cfblk4/2
  cfblk5/1 -> cfblk7/1

== system sampleModel20/cfblk96/cfblk5/cfblk4/cfblk11 ==
  cfblk1 : Inport
  cfblk5 : Inport  Port=2
  cfblk6 : Inport  Port=3
  cfblk3 : Sum  Inputs=+
  cfblk4 : MinMax  Function=max
  cfblk2 : Outport
  cfblk7 : Outport  Port=2
  wires:
  cfblk1/1 -> cfblk4/1
  cfblk3/1 -> cfblk2/1
  cfblk6/1 -> cfblk3/1
  cfblk4/1 -> cfblk7/1

== system sampleModel20/cfblk96/cfblk5/cfblk4/cfblk9 ==
  cfblk1 : Inport
  cfblk7 : Inport  Port=2
  cfblk8 : Inport  Port=3
  cfblk9 : Inport  Port=4
  cfblk3 : Sum  Inputs=+-
  cfblk4 : Signum
  cfblk5 : Sin  TimeSource=Use external signal  SampleTime=0
  cfblk6 : Polyval  Coefs=[ +2.081618890e-019, -1.441693666e-014, +4.719686976e-010, -8.536869453e-006, +1.621573104e-001, -8.087801117e+001 ]
  cfblk2 : Outport
  wires:
  cfblk5/1 -> cfblk3/1
  cfblk9/1 -> cfblk6/1
  cfblk1/1 -> cfblk5/1
  cfblk8/1 -> cfblk2/1
  cfblk7/1 -> cfblk4/1
  cfblk4/1 -> cfblk3/2

== system sampleModel20/cfblk96/cfblk5/cfblk6/cfblk5 ==
  cfblk1 : Inport
  cfblk8 : Inport  Port=2
  cfblk9 : Inport  Port=3
  cfblk10 : Inport  Port=4
  cfblk11 : Inport  Port=5
  cfblk3 : simulink/Math Operations/Slider Gain  gain=1  low=0  high=2
  cfblk4 : Sum  Inputs=--
  cfblk5 : Sum  Inputs=+-
  cfblk6 : Trigonometry
  cfblk7 : Polyval  Coefs=[ +2.081618890e-019, -1.441693666e-014, +4.719686976e-010, -8.536869453e-006, +1.621573104e-001, -8.087801117e+001 ]
  cfblk2 : Outport
  cfblk12 : Outport  Port=2
  wires:
  cfblk11/1 -> cfblk3/1
  cfblk3/1 -> cfblk7/1
  cfblk1/1 -> cfblk5/1
  cfblk6/1 -> cfblk4/1
  cfblk5/1 -> cfblk6/1
  cfblk7/1 -> cfblk4/2
  cfblk8/1 -> cfblk12/1
  cfblk4/1 -> cfblk2/1
  cfblk10/1 -> cfblk5/2

== system sampleModel20/cfblk96/cfblk5/cfblk6/cfblk6 ==
  cfblk1 : Inport
  cfblk9 : Inport  Port=2
  cfblk10 : Inport  Port=3
  cfblk11 : Inport  Port=4
  cfblk12 : Inport  Port=5
  cfblk13 : Inport  Port=6
  cfblk14 : Inport  Port=7
  cfblk3 : Math  Operator=rem  SaturateOnIntegerOverflow=on
  cfblk4 : Sqrt  Operator=rSqrt  AlgorithmType=Newton-Raphson  SaturateOnIntegerOverflow=on
  cfblk5 : simulink/Math Operations/Slider Gain  gain=1  low=0  high=2
  cfblk6 : Assignment  DiagnosticForDimensions=Warning  IndexOptions=Index vector (dialog)  Indices=1  OutputSizes=1
  cfblk7 : Product  Inputs=*
  cfblk8 : Sum  Inputs=|++
  cfblk2 : Outport
  wires:
  cfblk13/1 -> cfblk3/1
  cfblk10/1 -> cfblk3/2
  cfblk14/1 -> cfblk6/1
  cfblk1/1 -> cfblk2/1
  cfblk5/1 -> cfblk7/1
  cfblk6/1 -> cfblk4/1
  cfblk11/1 -> cfblk6/2
  cfblk12/1 -> cfblk8/1
  cfblk3/1 -> cfblk8/2
  cfblk9/1 -> cfblk5/1

== system sampleModel20/cfblk96/cfblk5/cfblk6/cfblk7 ==
  cfblk1 : Inport
  cfblk5 : Inport  Port=2
  cfblk6 : Inport  Port=3
  cfblk7 : Inport  Port=4
  cfblk3 : simulink/Math Operations/Slider Gain  gain=1  low=0  high=2
  cfblk4 : DotProduct  InputSameDT=on  OutDataTypeStr=Inherit: Inherit via internal rule
  cfblk2 : Outport
  wires:
  cfblk5/1 -> cfblk4/1
  cfblk1/1 -> cfblk4/2
  cfblk4/1 -> cfblk3/1
  cfblk7/1 -> cfblk2/1

== system sampleModel20/cfblk96/cfblk5/cfblk7/cfblk6 ==
  cfblk1 : Inport
  cfblk8 : Inport  Port=2
  cfblk9 : Inport  Port=3
  cfblk10 : Inport  Port=4
  cfblk11 : Inport  Port=5
  cfblk12 : Inport  Port=6
  cfblk13 : Inport  Port=7
  cfblk14 : Inport  Port=8
  cfblk3 : Sqrt  SaturateOnIntegerOverflow=on
  cfblk4 : Squeeze
  cfblk5 : Rounding
  cfblk6 : Sum  Inputs=|++
  cfblk7 : Product  Inputs=*
  cfblk2 : Outport
  wires:
  cfblk12/1 -> cfblk3/1
  cfblk14/1 -> cfblk4/1
  cfblk7/1 -> cfblk2/1
  cfblk8/1 -> cfblk7/1
  cfblk13/1 -> cfblk5/1
  cfblk1/1 -> cfblk6/1
  cfblk9/1 -> cfblk6/2

== system sampleModel20/cfblk96/cfblk5/cfblk7/cfblk7 ==
  cfblk1 : Inport
  cfblk11 : Inport  Port=2
  cfblk12 : Inport  Port=3
  cfblk13 : Inport  Port=4
  cfblk14 : Inport  Port=5
  cfblk15 : Inport  Port=6
  cfblk10 : Sin  TimeSource=Use external signal  SampleTime=0
  cfblk3 : Product
  cfblk4 : Rounding
  cfblk5 : simulink/Math Operations/Slider Gain  gain=1  low=0  high=2
  cfblk6 : Product  Inputs=**
  cfblk7 : simulink/Math Operations/Slider Gain  gain=1  low=0  high=2
  cfblk8 : Sqrt  Operator=rSqrt  AlgorithmType=Newton-Raphson  SaturateOnIntegerOverflow=on
  cfblk9 : Product  Inputs=**
  cfblk2 : Outport
  cfblk16 : Outport  Port=2
  wires:
  cfblk13/1 -> cfblk5/1
  cfblk15/1 -> cfblk9/1
  cfblk12/1 -> cfblk16/1
  cfblk14/1 -> cfblk6/1
  cfblk10/1 -> cfblk3/1
  cfblk6/1 -> cfblk4/1
  cfblk5/1 -> cfblk3/2
  cfblk1/1 -> cfblk7/1
  cfblk4/1 -> cfblk9/2
  cfblk11/1 -> cfblk6/2
  cfblk7/1 -> cfblk2/1
  cfblk3/1 -> cfblk8/1
  cfblk9/1 -> cfblk10/1

== system sampleModel20/cfblk96/cfblk5/cfblk8/cfblk6 ==
  cfblk1 : Inport
  cfblk5 : Inport  Port=2
  cfblk6 : Inport  Port=3
  cfblk7 : Inport  Port=4
  cfblk8 : Inport  Port=5
  cfblk9 : Inport  Port=6
  cfblk10 : Inport  Port=7
  cfblk3 : Product
  cfblk4 : Rounding
  cfblk2 : Outport
  cfblk11 : Outport  Port=2
  cfblk12 : Outport  Port=3
  wires:
  cfblk8/1 -> cfblk4/1
  cfblk5/1 -> cfblk12/1
  cfblk6/1 -> cfblk11/1
  cfblk9/1 -> cfblk3/1
  cfblk1/1 -> cfblk3/2
  cfblk3/1 -> cfblk2/1

== system sampleModel20/cfblk96/cfblk5/cfblk8/cfblk7 ==
  cfblk1 : Inport
  cfblk6 : Inport  Port=2
  cfblk7 : Inport  Port=3
  cfblk8 : Inport  Port=4
  cfblk9 : Inport  Port=5
  cfblk3 : Abs
  cfblk4 : Polyval  Coefs=[ +2.081618890e-019, -1.441693666e-014, +4.719686976e-010, -8.536869453e-006, +1.621573104e-001, -8.087801117e+001 ]
  cfblk5 : Abs
  cfblk2 : Outport
  wires:
  cfblk1/1 -> cfblk4/1
  cfblk8/1 -> cfblk5/1
  cfblk9/1 -> cfblk3/1
  cfblk5/1 -> cfblk2/1

== system sampleModel20/cfblk96/cfblk5/cfblk8/cfblk8 ==
  cfblk1 : Inport
  cfblk11 : Inport  Port=2
  cfblk12 : Inport  Port=3
  cfblk13 : Inport  Port=4
  cfblk14 : Inport  Port=5
  cfblk10 : Trigonometry
  cfblk3 : Delay  SampleTime=1
  cfblk4 : DotProduct  InputSameDT=on  OutDataTypeStr=Inherit: Inherit via internal rule
  cfblk5 : Gain  Gain=[310661570.017494]
  cfblk6 : ComplexToMagnitudeAngle
  cfblk7 : Trigonometry
  cfblk8 : Product  Inputs=*
  cfblk9 : Trigonometry
  cfblk2 : Outport
  cfblk15 : Outport  Port=2
  cfblk16 : Outport  Port=3
  wires:
  cfblk3/1 -> cfblk8/1
  cfblk1/1 -> cfblk9/1
  cfblk5/1 -> cfblk3/1
  cfblk11/1 -> cfblk10/1
  cfblk10/1 -> cfblk15/1
  cfblk8/1 -> cfblk16/1
  cfblk4/1 -> cfblk6/1
  cfblk9/1 -> cfblk4/1
  cfblk6/1 -> cfblk7/1
  cfblk14/1 -> cfblk5/1
  cfblk6/2 -> cfblk2/1
  cfblk12/1 -> cfblk4/2

== system sampleModel20/cfblk96/cfblk5/cfblk8/cfblk9 ==
  cfblk1 : Inport
  cfblk9 : Inport  Port=2
  cfblk10 : Inport  Port=3
  cfblk11 : Inport  Port=4
  cfblk12 : Inport  Port=5
  cfblk13 : Inport  Port=6
  cfblk14 : Inport  Port=7
  cfblk15 : Inport  Port=8
  cfblk3 : Sin  TimeSource=Use external signal  SampleTime=0
  cfblk4 : simulink/Math Operations/Slider Gain  gain=1  low=0  high=2
  cfblk5 : UnaryMinus
  cfblk6 : Rounding
  cfblk7 : Trigonometry
  cfblk8 : Product  Inputs=*
  cfblk2 : Outport
  cfblk16 : Outport  Port=2
  cfblk17 : Outport  Port=3
  wires:
  cfblk9/1 -> cfblk17/1
  cfblk4/1 -> cfblk6/1
  cfblk15/1 -> cfblk8/1
  cfblk7/1 -> cfblk5/1
  cfblk8/1 -> cfblk2/1
  cfblk13/1 -> cfblk4/1
  cfblk3/1 -> cfblk16/1
  cfblk1/1 -> cfblk7/1
  cfblk6/1 -> cfblk3/1

== system sampleModel20/cfblk96/cfblk6/cfblk5/cfblk10 ==
  cfblk1 : Inport
  cfblk7 : Inport  Port=2
  cfblk8 : Inport  Port=3
  cfblk3 : simulink/Math Operations/Slider Gain  gain=1  low=0  high=2
  cfblk4 : Polyval  Coefs=[ +2.081618890e-019, -1.441693666e-014, +4.719686976e-010, -8.536869453e-006, +1.621573104e-001, -8.087801117e+001 ]
  cfblk5 : Sqrt  Operator=rSqrt  AlgorithmType=Newton-Raphson  SaturateOnIntegerOverflow=on
  cfblk6 : simulink/Math Operations/Slider Gain  gain=1  low=0  high=2
  cfblk2 : Outport
  wires:
  cfblk6/1 -> cfblk4/1
  cfblk4/1 -> cfblk3/1
  cfblk1/1 -> cfblk6/1
  cfblk8/1 -> cfblk2/1
  cfblk7/1 -> cfblk5/1

== system sampleModel20/cfblk96/cfblk6/cfblk5/cfblk11 ==
  cfblk1 : Inport
  cfblk5 : Inport  Port=2
  cfblk6 : Inport  Port=3
  cfblk7 : Inport  Port=4
  cfblk8 : Inport  Port=5
  cfblk9 : Inport  Port=6
  cfblk10 : Inport  Port=7
  cfblk3 : Trigonometry
  cfblk4 : simulink/Math Operations/MinMax Running Resettable  Function=min  vinit=0.0
  cfblk2 : Outport
  cfblk11 : Outport  Port=2
  wires:
  cfblk10/1 -> cfblk2/1
  cfblk9/1 -> cfblk3/1
  cfblk8/1 -> cfblk4/1
  cfblk3/1 -> cfblk4/2
  cfblk7/1 -> cfblk11/1

== system sampleModel20/cfblk96/cfblk6/cfblk5/cfblk12 ==
  cfblk1 : Inport
  cfblk6 : Inport  Port=2
  cfblk7 : Inport  Port=3
  cfblk10 : Delay  SampleTime=1
  cfblk3 : Polyval  Coefs=[ +2.081618890e-019, -1.441693666e-014, +4.719686976e-010, -8.536869453e-006, +1.621573104e-001, -8.087801117e+001 ]
  cfblk4 : Product
  cfblk5 : Sum  Inputs=-+
  cfblk2 : Outport
  cfblk8 : Outport  Port=2
  cfblk9 : Outport  Port=3
  wires:
  cfblk7/1 -> cfblk4/1
  cfblk3/1 -> cfblk4/2
  cfblk1/1 -> cfblk2/1, cfblk5/2
  cfblk6/1 -> cfblk5/1
  cfblk5/1 -> cfblk9/1, cfblk8/1
  cfblk4/1 -> cfblk10/1
  cfblk10/1 -> cfblk3/1

== system sampleModel20/cfblk96/cfblk6/cfblk5/cfblk13 ==
  cfblk1 : Inport
  cfblk7 : Inport  Port=2
  cfblk8 : Inport  Port=3
  cfblk9 : Inport  Port=4
  cfblk10 : Inport  Port=5
  cfblk11 : Inport  Port=6
  cfblk3 : Trigonometry
  cfblk4 : DotProduct  InputSameDT=on  OutDataTypeStr=Inherit: Inherit via internal rule
  cfblk5 : Product
  cfblk6 : Sum  Inputs=+-
  cfblk2 : Outport
  cfblk12 : Outport  Port=2
  cfblk13 : Outport  Port=3
  cfblk14 : Outport  Port=4
  cfblk15 : Outport  Port=5
  wires:
  cfblk8/1 -> cfblk2/1, cfblk6/1
  cfblk10/1 -> cfblk12/1
  cfblk3/1 -> cfblk4/1
  cfblk7/1 -> cfblk14/1
  cfblk11/1 -> cfblk4/2
  cfblk6/1 -> cfblk15/1
  cfblk1/1 -> cfblk5/1
  cfblk9/1 -> cfblk5/2
  cfblk5/1 -> cfblk3/1
  cfblk4/1 -> cfblk13/1, cfblk6/2

== system sampleModel20/cfblk96/cfblk6/cfblk5/cfblk14 ==
  cfblk1 : Inport
  cfblk5 : Inport  Port=2
  cfblk6 : Inport  Port=3
  cfblk7 : Inport  Port=4
  cfblk3 : Reshape
  cfblk4 : simulink/Math Operations/MinMax Running Resettable  Function=min  vinit=0.0
  cfblk2 : Outport
  wires:
  cfblk3/1 -> cfblk4/1
  cfblk5/1 -> cfblk4/2
  cfblk1/1 -> cfblk3/1
  cfblk6/1 -> cfblk2/1

== system sampleModel20/cfblk96/cfblk7/cfblk6/cfblk10 ==
  cfblk1 : Inport
  cfblk8 : Inport  Port=2
  cfblk9 : Inport  Port=3
  cfblk10 : Inport  Port=4
  cfblk11 : Inport  Port=5
  cfblk12 : Inport  Port=6
  cfblk13 : Inport  Port=7
  cfblk14 : Inport  Port=8
  cfblk3 : Gain  Gain=[-237050810.076699]
  cfblk4 : Trigonometry
  cfblk5 : Abs
  cfblk6 : Sum  Inputs=+
  cfblk7 : Reshape
  cfblk2 : Outport
  cfblk15 : Outport  Port=2
  cfblk16 : Outport  Port=3
  wires:
  cfblk10/1 -> cfblk7/1
  cfblk7/1 -> cfblk5/1
  cfblk14/1 -> cfblk2/1
  cfblk4/1 -> cfblk6/1
  cfblk5/1 -> cfblk3/1
  cfblk3/1 -> cfblk4/1
  cfblk12/1 -> cfblk16/1
  cfblk6/1 -> cfblk15/1

== system sampleModel20/cfblk96/cfblk7/cfblk6/cfblk11 ==
  cfblk1 : Inport
  cfblk7 : Inport  Port=2
  cfblk8 : Inport  Port=3
  cfblk9 : Inport  Port=4
  cfblk10 : Inport  Port=5
  cfblk11 : Inport  Port=6
  cfblk12 : Inport  Port=7
  cfblk16 : Delay  SampleTime=1
  cfblk3 : Squeeze
  cfblk4 : Gain  Gain=[-261208180.405835]
  cfblk5 : PermuteDimensions
  cfblk6 : DotProduct  InputSameDT=on  OutDataTypeStr=Inherit: Inherit via internal rule
  cfblk2 : Outport
  cfblk13 : Outport  Port=2
  cfblk14 : Outport  Port=3
  cfblk15 : Outport  Port=4
  wires:
  cfblk4/1 -> cfblk5/1
  cfblk7/1 -> cfblk3/1
  cfblk1/1 -> cfblk2/1
  cfblk9/1 -> cfblk13/1
  cfblk3/1 -> cfblk15/1
  cfblk12/1 -> cfblk14/1
  cfblk11/1 -> cfblk6/1
  cfblk10/1 -> cfblk6/2
  cfblk5/1 -> cfblk16/1
  cfblk16/1 -> cfblk4/1

== system sampleModel20/cfblk96/cfblk7/cfblk6/cfblk12 ==
  cfblk1 : Inport
  cfblk4 : Inport  Port=2
  cfblk5 : Inport  Port=3
  cfblk6 : Inport  Port=4
  cfblk3 : MinMax  Function=max
  cfblk2 : Outport
  cfblk7 : Outport  Port=2
  cfblk8 : Outport  Port=3
  wires:
  cfblk6/1 -> cfblk2/1
  cfblk3/1 -> cfblk8/1
  cfblk4/1 -> cfblk7/1
  cfblk5/1 -> cfblk3/1

== system sampleModel20/cfblk96/cfblk7/cfblk6/cfblk13 ==
  cfblk1 : Inport
  cfblk8 : Inport  Port=2
  cfblk9 : Inport  Port=3
  cfblk10 : Inport  Port=4
  cfblk11 : Inport  Port=5
  cfblk3 : Rounding
  cfblk4 : Assignment  DiagnosticForDimensions=Warning  IndexOptions=Index vector (dialog)  Indices=1  OutputSizes=1
  cfblk5 : simulink/Math Operations/MinMax Running Resettable  Function=min  vinit=0.0
  cfblk6 : Rounding
  cfblk7 : Sin  TimeSource=Use external signal  SampleTime=0
  cfblk2 : Outport
  wires:
  cfblk7/1 -> cfblk6/1
  cfblk8/1 -> cfblk7/1
  cfblk6/1 -> cfblk2/1
  cfblk9/1 -> cfblk4/1
  cfblk11/1 -> cfblk5/1
  cfblk1/1 -> cfblk3/1
  cfblk3/1 -> cfblk5/2
  cfblk5/1 -> cfblk4/2

== system sampleModel20/cfblk96/cfblk7/cfblk6/cfblk8 ==
  cfblk1 : Inport
  cfblk6 : Inport  Port=2
  cfblk7 : Inport  Port=3
  cfblk8 : Inport  Port=4
  cfblk9 : Inport  Port=5
  cfblk3 : Sqrt  SaturateOnIntegerOverflow=on
  cfblk4 : Gain  Gain=[675853537.607548]
  cfblk5 : Sin  TimeSource=Use external signal  SampleTime=0
  cfblk2 : Outport
  wires:
  cfblk1/1 -> cfblk5/1
  cfblk6/1 -> cfblk2/1
  cfblk3/1 -> cfblk4/1
  cfblk7/1 -> cfblk3/1

== system sampleModel20/cfblk96/cfblk7/cfblk6/cfblk9 ==
  cfblk1 : Inport
  cfblk9 : Inport  Port=2
  cfblk10 : Inport  Port=3
  cfblk11 : Inport  Port=4
  cfblk12 : Inport  Port=5
  cfblk13 : Inport  Port=6
  cfblk14 : Inport  Port=7
  cfblk15 : Inport  Port=8
  cfblk17 : Delay  SampleTime=1
  cfblk3 : Rounding
  cfblk4 : Math  SaturateOnIntegerOverflow=on
  cfblk5 : MinMax  Function=max  Inputs=2
  cfblk6 : Assignment  DiagnosticForDimensions=Warning  IndexOptions=Index vector (dialog)  Indices=1  OutputSizes=1
  cfblk7 : MinMax  Inputs=2
  cfblk8 : ComplexToMagnitudeAngle
  cfblk2 : Outport
  cfblk16 : Outport  Port=2
  wires:
  cfblk13/1 -> cfblk16/1
  cfblk11/1 -> cfblk5/1
  cfblk8/1 -> cfblk5/2
  cfblk15/1 -> cfblk8/1
  cfblk10/1 -> cfblk6/1
  cfblk1/1 -> cfblk7/1
  cfblk3/1 -> cfblk6/2
  cfblk9/1 -> cfblk4/1
  cfblk4/1 -> cfblk7/2
  cfblk8/2 -> cfblk2/1
  cfblk6/1 -> cfblk17/1
  cfblk17/1 -> cfblk3/1

== system sampleModel20/cfblk96/cfblk7/cfblk7/cfblk10 ==
  cfblk1 : Inport
  cfblk8 : Inport  Port=2
  cfblk9 : Inport  Port=3
  cfblk10 : Inport  Port=4
  cfblk11 : Inport  Port=5
  cfblk3 : ComplexToMagnitudeAngle
  cfblk4 : DotProduct  InputSameDT=on  OutDataTypeStr=Inherit: Inherit via internal rule
  cfblk5 : Squeeze
  cfblk6 : Sum
  cfblk7 : Product
  cfblk2 : Outport
  cfblk12 : Outport  Port=2
  cfblk13 : Outport  Port=3
  wires:
  cfblk4/1 -> cfblk7/1
  cfblk5/1 -> cfblk6/1
  cfblk9/1 -> cfblk3/1
  cfblk1/1 -> cfblk5/1
  cfblk7/1 -> cfblk13/1
  cfblk11/1 -> cfblk12/1
  cfblk10/1 -> cfblk6/2
  cfblk3/1 -> cfblk7/2
  cfblk3/2 -> cfblk2/1
  cfblk8/1 -> cfblk4/1
  cfblk6/1 -> cfblk4/2

== system sampleModel20/cfblk96/cfblk7/cfblk7/cfblk11 ==
  cfblk1 : Inport
  cfblk10 : Inport  Port=2
  cfblk11 : Delay  SampleTime=1
  cfblk3 : Gain  Gain=[-676500443.205479]
  cfblk4 : DotProduct  InputSameDT=on  OutDataTypeStr=Inherit: Inherit via internal rule
  cfblk5 : Assignment  DiagnosticForDimensions=Warning  IndexOptions=Index vector (dialog)  Indices=1  OutputSizes=1
  cfblk6 : simulink/Math Operations/Slider Gain  gain=1  low=0  high=2
  cfblk7 : Reshape
  cfblk8 : Sqrt  Operator=rSqrt  AlgorithmType=Newton-Raphson  SaturateOnIntegerOverflow=on
  cfblk9 : simulink/Math Operations/Slider Gain  gain=1  low=0  high=2
  cfblk2 : Outport
  wires:
  cfblk5/1 -> cfblk7/1
  cfblk4/1 -> cfblk9/1
  cfblk6/1 -> cfblk4/1
  cfblk7/1 -> cfblk8/1
  cfblk9/1 -> cfblk2/1, cfblk5/2
  cfblk1/1 -> cfblk3/1
  cfblk3/1 -> cfblk4/2
  cfblk10/1 -> cfblk6/1
  cfblk8/1 -> cfblk11/1
  cfblk11/1 -> cfblk5/1

== system sampleModel20/cfblk96/cfblk7/cfblk8/cfblk9 ==
  cfblk1 : Inport
  cfblk8 : Inport  Port=2
  cfblk9 : Inport  Port=3
  cfblk10 : Inport  Port=4
  cfblk11 : Inport  Port=5
  cfblk12 : Inport  Port=6
  cfblk3 : PermuteDimensions
  cfblk4 : Reshape
  cfblk5 : Trigonometry
  cfblk6 : Sum  Inputs=|++
  cfblk7 : Product  Inputs=*
  cfblk2 : Outport
  cfblk13 : Outport  Port=2
  cfblk14 : Outport  Port=3
  wires:
  cfblk10/1 -> cfblk2/1
  cfblk7/1 -> cfblk3/1
  cfblk6/1 -> cfblk13/1
  cfblk11/1 -> cfblk4/1
  cfblk5/1 -> cfblk14/1
  cfblk4/1 -> cfblk5/1
  cfblk8/1 -> cfblk6/1
  cfblk9/1 -> cfblk6/2
  cfblk12/1 -> cfblk7/1

== system sampleModel20/cfblk97/cfblk3/cfblk10/cfblk6 ==
  cfblk1 : Inport
  cfblk7 : Inport  Port=2
  cfblk8 : Inport  Port=3
  cfblk9 : Inport  Port=4
  cfblk10 : Inport  Port=5
  cfblk11 : Inport  Port=6
  cfblk12 : Inport  Port=7
  cfblk13 : Inport  Port=8
  cfblk14 : Inport  Port=9
  cfblk15 : Inport  Port=10
  cfblk16 : Inport  Port=11
  cfblk3 : simulink/Discrete/Transfer Fcn Lead or Lag  PoleZ=0.95  ZeroZ=0.75  ICPrevOutput=0.0  ICPrevInput=0.0  DoSatur=off
      settings: SourceProductBaseCode=SL
  cfblk4 : Squeeze
  cfblk5 : Product  Inputs=**
  cfblk6 : Gain  Gain=[839312755.920593]
  cfblk2 : Outport
  wires:
  cfblk6/1 -> cfblk4/1
  cfblk14/1 -> cfblk3/1
  cfblk7/1 -> cfblk6/1
  cfblk3/1 -> cfblk5/1
  cfblk16/1 -> cfblk5/2
  cfblk15/1 -> cfblk2/1
